simulink model "QuadDynamics"  (R2017b)
settings: Solver=FixedStepAuto  StartTime=0.0  StopTime=10  FixedStep=0.01  RelTol=1e-3
InitFcn:
  | glob
values from neighbouring files (symbols this model uses):
  Earth_g = 9.8    [constant.m]
  UAV_aaa = inv([UAV_kf UAV_kf UAV_kf UAV_kf ... (first row only)    [constant.m]
  UAV_Ixx = 19.688e-3    (= 0.019688)    [constant.m]
  UAV_Iyy = 19.688e-3    (= 0.019688)    [constant.m]
  UAV_Izz = 3.938e-2    (= 0.03938)    [constant.m]
  UAV_kdphi = 0    [constant.m]
  UAV_kdpsai = 0    [constant.m]
  UAV_kdtheta = UAV_kdphi    (= 0)    [constant.m]
  UAV_kdx = 0    [constant.m]
  UAV_kdy = 0    [constant.m]
  UAV_kdz = 0    [constant.m]
  UAV_kipsai = 0    [constant.m]
  UAV_kix = 0    [constant.m]
  UAV_kiy = 0    [constant.m]
  UAV_kiz = 0    [constant.m]
  UAV_kpphi = 0    [constant.m]
  UAV_kppsai = 0    [constant.m]
  UAV_kptheta = UAV_kpphi    (= 0)    [constant.m]
  UAV_kpx = 0    [constant.m]
  UAV_kpy = 0    [constant.m]
  UAV_kpz = 0    [constant.m]
  UAV_L = 0.25    [constant.m]
  UAV_m = 0.75    [constant.m]
  UAV_xf = 3    [constant.m]
  UAV_yf = 4    [constant.m]
  UAV_zf = 5    [constant.m]
settings Model: Creator=root  LastModifiedBy=KingBoy
settings CodeAppCC: StateflowObjectComments=on

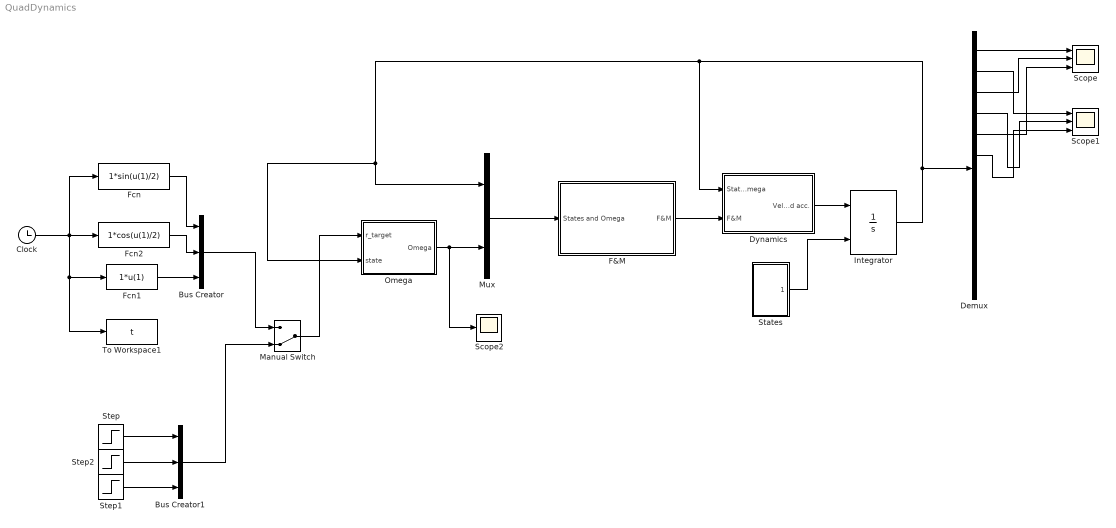
== system QuadDynamics ==
  Bus Creator : BusCreator  Inputs=3
  Bus Creator1 : BusCreator  Inputs=3
  Clock : Clock
  Demux : Demux  Outputs=12
  Dynamics : Subsystem
  F&M : Subsystem
  Fcn : Fcn  Expr=1*sin(u(1)/2)
  Fcn1 : Fcn  Expr=1*u(1)
  Fcn2 : Fcn  Expr=1*cos(u(1)/2)
  Integrator : Integrator  InitialConditionSource=external
  Manual Switch : ManualSwitch  CurrentSetting=0
  Mux : Mux  Inputs=2
  Omega : Subsystem
  Scope : Scope  NumInputPorts=3
  Scope1 : Scope  NumInputPorts=3
  Scope2 : Scope
  States : Subsystem
  Step : Step  Time=0  After=UAV_xf  SampleTime=0
  Step1 : Step  Time=0  After=UAV_zf  SampleTime=0
  Step2 : Step  Time=0  After=UAV_yf  SampleTime=0
  To Workspace1 : ToWorkspace  VariableName=t  SampleTime=-1
      settings: Save2DSignal=2-D array (concatenate along first dimension)
  wires:
  F&M/1(F&M) -> Dynamics/2(F&M)
  Integrator/1 -> Demux/1, Omega/2(state), Mux/1, Dynamics/1(States and Omega)
  Demux/5 -> Scope/3
  States/1("States ") -> Integrator/2
  Omega/1("Omega ") -> Scope2/1, Mux/2
  Mux/1 -> F&M/1(States and Omega)
  Dynamics/1("Velocity and acc. ") -> Integrator/1
  Demux/1 -> Scope/1
  Demux/3 -> Scope/2
  Demux/4 -> Scope1/2
  Demux/6 -> Scope1/3
  Fcn1/1 -> Bus Creator/3
  Clock/1 -> To Workspace1/1, Fcn1/1, Fcn/1, Fcn2/1
  Fcn/1 -> Bus Creator/1
  Fcn2/1 -> Bus Creator/2
  Bus Creator/1 -> Manual Switch/1
  Step2/1 -> Bus Creator1/2
  Step/1 -> Bus Creator1/1
  Bus Creator1/1 -> Manual Switch/2
  Step1/1 -> Bus Creator1/3
  Manual Switch/1 -> Omega/1(r_target)
  Demux/2 -> Scope1/1

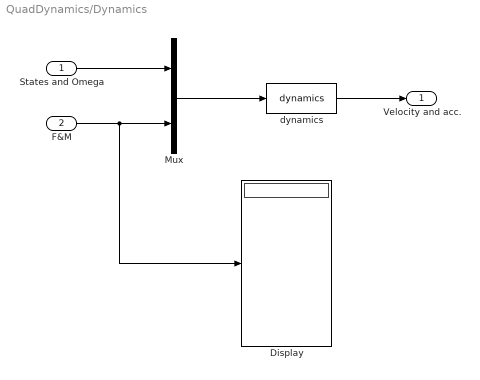
== system QuadDynamics/Dynamics ==
  States and Omega : Inport
  F&M : Inport  Port=2
  Display : Display
  Mux : Mux  Inputs=2
  dynamics : MATLABFcn  MATLABFcn=dynamics  OutputDimensions=12
  "Velocity and acc. " : Outport
  wires:
  Mux/1 -> dynamics/1
  F&M/1 -> Display/1, Mux/2
  States and Omega/1 -> Mux/1
  dynamics/1 -> "Velocity and acc. "/1

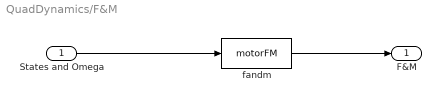
== system QuadDynamics/F&M ==
  States and Omega : Inport
  fandm : MATLABFcn  MATLABFcn=motorFM  OutputDimensions=8
  F&M : Outport
  wires:
  fandm/1 -> F&M/1
  States and Omega/1 -> fandm/1

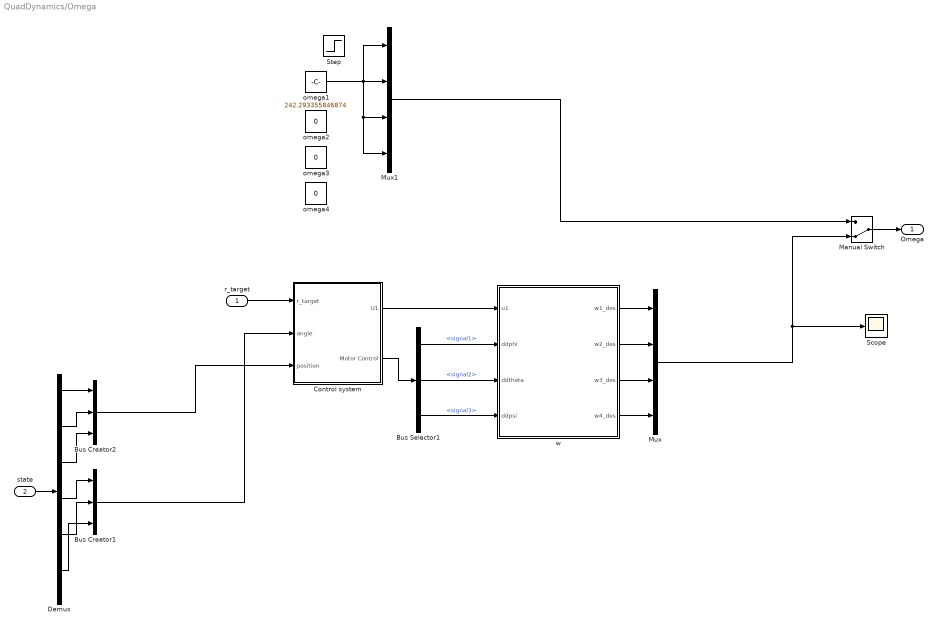
== system QuadDynamics/Omega ==
  r_target : Inport
  state : Inport  Port=2
  Bus Creator1 : BusCreator  Inputs=3
  Bus Creator2 : BusCreator  Inputs=3
  Bus Selector1 : BusSelector  OutputSignals=signal1,signal2,signal3
  Control system : Subsystem
  Demux : Demux  Outputs=12
  Manual Switch : ManualSwitch  CurrentSetting=0
  Mux : Mux
  Mux1 : Mux
  Scope : Scope
  Step : Step  Time=0  After=3  SampleTime=0
  omega1 : Constant  Value=242.293355846874
  omega2 : Constant  Value=0
  omega3 : Constant  Value=0
  omega4 : Constant  Value=0
  w : Subsystem
  "Omega " : Outport
  wires:
  Bus Selector1/3 -> w/4(ddpsi)  "<signal3>"
  Bus Selector1/2 -> w/3(ddtheta)  "<signal2>"
  Bus Selector1/1 -> w/2(ddphi)  "<signal1>"
  Control system/1(U1) -> w/1(u1)
  Control system/2(Motor Control) -> Bus Selector1/1
  w/1(w1_des) -> Mux/1
  w/2(w2_des) -> Mux/2
  w/3(w3_des) -> Mux/3
  w/4(w4_des) -> Mux/4
  r_target/1 -> Control system/1(r_target)
  state/1 -> Demux/1
  Demux/1 -> Bus Creator2/1
  Demux/3 -> Bus Creator2/2
  Demux/5 -> Bus Creator2/3
  Bus Creator2/1 -> Control system/3(position)
  Bus Creator1/1 -> Control system/2(angle)
  Manual Switch/1 -> "Omega "/1
  Mux1/1 -> Manual Switch/1
  Demux/7 -> Bus Creator1/1
  Demux/9 -> Bus Creator1/2
  Demux/11 -> Bus Creator1/3
  Mux/1 -> Scope/1, Manual Switch/2
  omega1/1 -> Mux1/3, Mux1/4, Mux1/2, Mux1/1

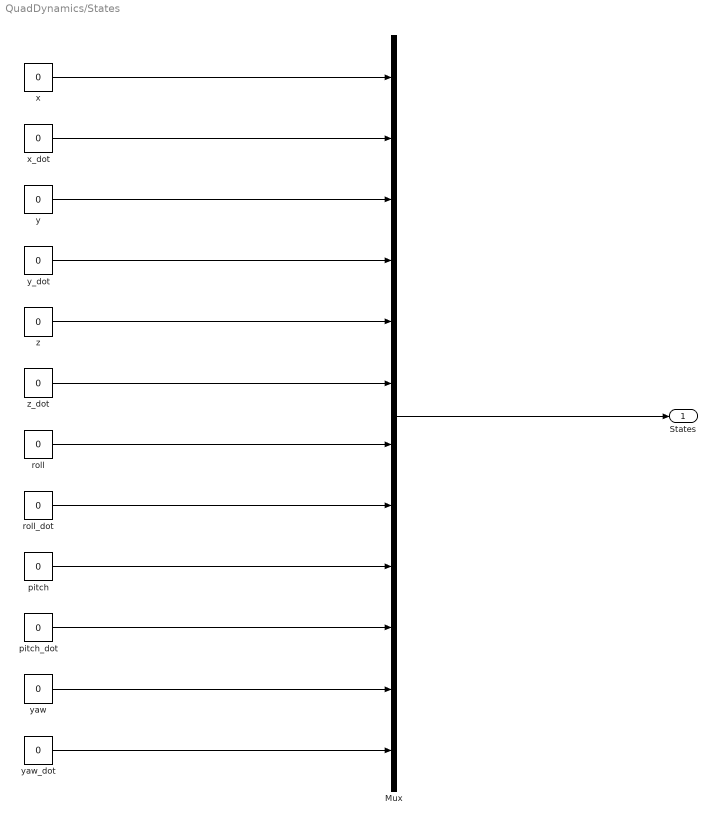
== system QuadDynamics/States ==
  Mux : Mux  Inputs=12
  pitch : Constant  Value=0
  pitch_dot : Constant  Value=0
  roll : Constant  Value=0
  roll_dot : Constant  Value=0
  x : Constant  Value=0
  x_dot : Constant  Value=0
  y : Constant  Value=0
  y_dot : Constant  Value=0
  yaw : Constant  Value=0
  yaw_dot : Constant  Value=0
  z : Constant  Value=0
  z_dot : Constant  Value=0
  "States " : Outport
  wires:
  y/1 -> Mux/3
  z/1 -> Mux/5
  z_dot/1 -> Mux/6
  x/1 -> Mux/1
  pitch_dot/1 -> Mux/10
  x_dot/1 -> Mux/2
  roll/1 -> Mux/7
  yaw/1 -> Mux/11
  y_dot/1 -> Mux/4
  pitch/1 -> Mux/9
  roll_dot/1 -> Mux/8
  yaw_dot/1 -> Mux/12
  Mux/1 -> "States "/1

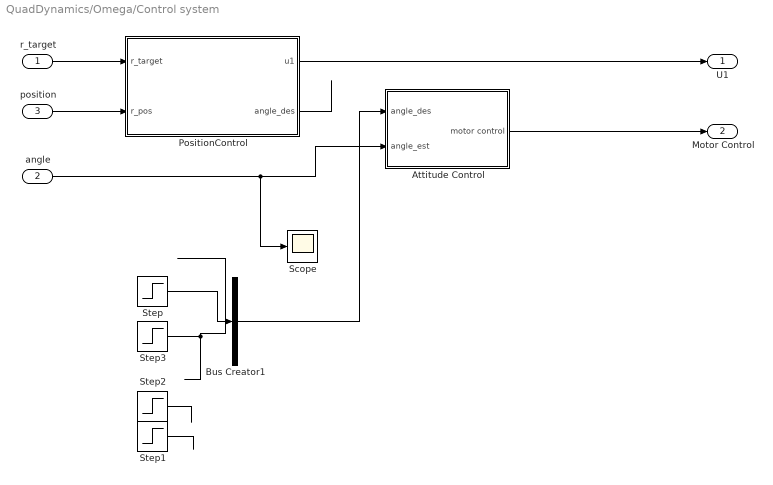
== system QuadDynamics/Omega/Control system ==
  r_target : Inport
  angle : Inport  Port=2
  position : Inport  Port=3
  Attitude Control : Subsystem
  Bus Creator1 : BusCreator  Inputs=3
  PositionControl : Subsystem
  Scope : Scope
  Step : Step  Time=0  After=pi/6  SampleTime=0
  Step1 : Step  Time=0  After=UAV_zf  SampleTime=0
  Step2 : Step  Time=0  After=UAV_yf  SampleTime=0
  Step3 : Step  Time=0  After=0  SampleTime=0
  U1 : Outport
  Motor Control : Outport  Port=2
  wires:
  PositionControl/2(angle_des) -> ?
  angle/1 -> Scope/1, Attitude Control/2(angle_est)
  PositionControl/1(u1) -> U1/1
  Attitude Control/1(motor control) -> Motor Control/1
  position/1 -> PositionControl/2(r_pos)
  r_target/1 -> PositionControl/1(r_target)
  Bus Creator1/1 -> Attitude Control/1(angle_des)
  Step1/1 -> ?
  Step/1 -> Bus Creator1/2
  Step2/1 -> ?
  Step3/1 -> ?

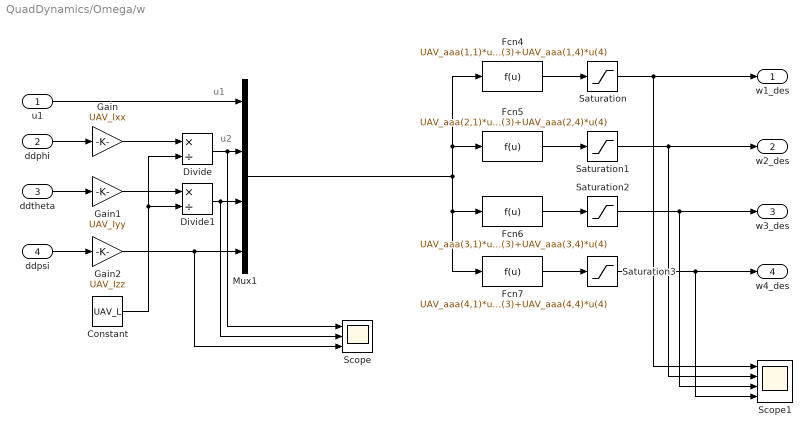
== system QuadDynamics/Omega/w ==
  note: u2
  note: u1
  u1 : Inport
  ddphi : Inport  Port=2
  ddtheta : Inport  Port=3
  ddpsi : Inport  Port=4
  Constant : Constant  Value=UAV_L
  Divide : Product  Inputs=*/
  Divide1 : Product  Inputs=*/
  Fcn4 : Fcn  Expr=UAV_aaa(1,1)*u(1)+UAV_aaa(1,2)*u(2)+UAV_aaa(1,3)*u(3)+UAV_aaa(1,4)*u(4)
  Fcn5 : Fcn  Expr=UAV_aaa(2,1)*u(1)+UAV_aaa(2,2)*u(2)+UAV_aaa(2,3)*u(3)+UAV_aaa(2,4)*u(4)
  Fcn6 : Fcn  Expr=UAV_aaa(3,1)*u(1)+UAV_aaa(3,2)*u(2)+UAV_aaa(3,3)*u(3)+UAV_aaa(3,4)*u(4)
  Fcn7 : Fcn  Expr=UAV_aaa(4,1)*u(1)+UAV_aaa(4,2)*u(2)+UAV_aaa(4,3)*u(3)+UAV_aaa(4,4)*u(4)
  Gain : Gain  Gain=UAV_Ixx
  Gain1 : Gain  Gain=UAV_Iyy
  Gain2 : Gain  Gain=UAV_Izz
  Mux1 : Mux
  Saturation{,1..3} (4 alike) : Saturate  UpperLimit=(9000*2*pi/60)^2  LowerLimit=0
  Scope : Scope  NumInputPorts=3
  Scope1 : Scope  NumInputPorts=4
  w1_des : Outport
  w2_des : Outport  Port=2
  w3_des : Outport  Port=3
  w4_des : Outport  Port=4
  wires:
  u1/1 -> Mux1/1
  ddphi/1 -> Gain/1
  ddpsi/1 -> Gain2/1
  ddtheta/1 -> Gain1/1
  Fcn4/1 -> Saturation/1
  Fcn6/1 -> Saturation2/1
  Fcn7/1 -> Saturation3/1
  Saturation/1 -> Scope1/1, w1_des/1
  Saturation1/1 -> Scope1/2, w2_des/1
  Saturation2/1 -> Scope1/3, w3_des/1
  Saturation3/1 -> Scope1/4, w4_des/1
  Divide/1 -> Scope/1, Mux1/2
  Gain/1 -> Divide/1
  Constant/1 -> Divide1/2, Divide/2
  Divide1/1 -> Scope/2, Mux1/3
  Gain2/1 -> Scope/3, Mux1/4
  Gain1/1 -> Divide1/1
  Fcn5/1 -> Saturation1/1
  Mux1/1 -> Fcn7/1, Fcn6/1, Fcn5/1, Fcn4/1

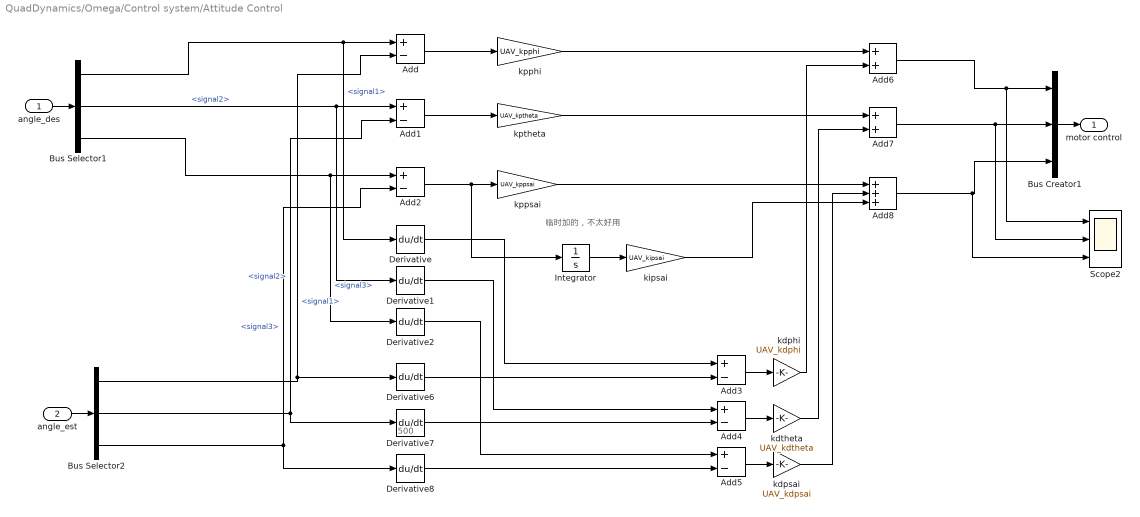
== system QuadDynamics/Omega/Control system/Attitude Control ==
  note: 临时加的，不太好用
  note: 500
  angle_des : Inport
  angle_est : Inport  Port=2
  Add{,1..5} (6 alike) : Sum  Inputs=+-
  Add6 : Sum
  Add7 : Sum
  Add8 : Sum  Inputs=+++
  Bus Creator1 : BusCreator  Inputs=3
  Bus Selector1 : BusSelector  OutputSignals=signal1,signal2,signal3
  Bus Selector2 : BusSelector  OutputSignals=signal1,signal2,signal3
  Derivative{,1..2,6..8} (6 alike) : Derivative  CoefficientInTFapproximation=500
  Integrator : Integrator
  Scope2 : Scope  NumInputPorts=3
  kdphi : Gain  Gain=UAV_kdphi
  kdpsai : Gain  Gain=UAV_kdpsai
  kdtheta : Gain  Gain=UAV_kdtheta
  kipsai : Gain  Gain=UAV_kipsai
  kpphi : Gain  Gain=UAV_kpphi
  kppsai : Gain  Gain=UAV_kppsai
  kptheta : Gain  Gain=UAV_kptheta
  motor control : Outport
  wires:
  Bus Selector1/1 -> Add/1, Derivative/1  "<signal1>"
  Bus Selector2/1 -> Add/2, Derivative6/1  "<signal1>"
  Add/1 -> kpphi/1
  Bus Selector1/2 -> Derivative1/1, Add1/1  "<signal2>"
  Bus Selector2/2 -> Add1/2, Derivative7/1  "<signal2>"
  Add1/1 -> kptheta/1
  Add2/1 -> Integrator/1, kppsai/1
  Bus Selector1/3 -> Derivative2/1, Add2/1  "<signal3>"
  Bus Selector2/3 -> Add2/2, Derivative8/1  "<signal3>"
  Add3/1 -> kdphi/1
  Add4/1 -> kdtheta/1
  Add5/1 -> kdpsai/1
  kpphi/1 -> Add6/1
  kdphi/1 -> Add6/2
  kptheta/1 -> Add7/1
  kdtheta/1 -> Add7/2
  kppsai/1 -> Add8/1
  kdpsai/1 -> Add8/2
  Derivative/1 -> Add3/1
  Derivative1/1 -> Add4/1
  Derivative2/1 -> Add5/1
  Derivative6/1 -> Add3/2
  Derivative7/1 -> Add4/2
  Derivative8/1 -> Add5/2
  angle_est/1 -> Bus Selector2/1
  angle_des/1 -> Bus Selector1/1
  Bus Creator1/1 -> motor control/1
  Add6/1 -> Scope2/1, Bus Creator1/1
  Add7/1 -> Scope2/2, Bus Creator1/2
  Add8/1 -> Scope2/3, Bus Creator1/3
  Integrator/1 -> kipsai/1
  kipsai/1 -> Add8/3

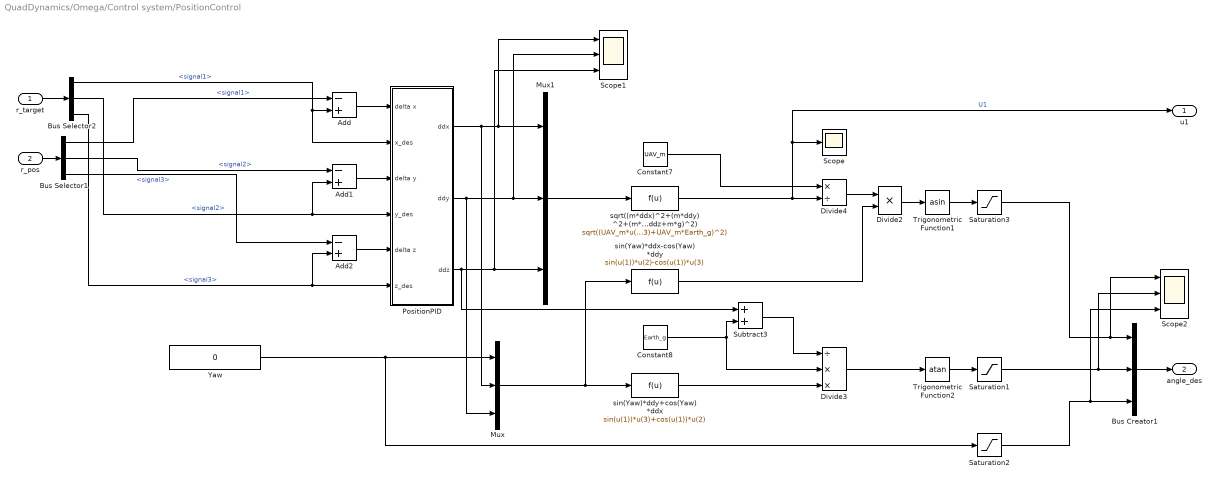
== system QuadDynamics/Omega/Control system/PositionControl ==
  r_target : Inport
  r_pos : Inport  Port=2
  Add : Sum  Inputs=-+
  Add1 : Sum  Inputs=-+
  Add2 : Sum  Inputs=-+
  Bus Creator1 : BusCreator  Inputs=3
  Bus Selector1 : BusSelector  OutputSignals=signal1,signal2,signal3
  Bus Selector2 : BusSelector  OutputSignals=signal1,signal2,signal3
  Constant7 : Constant  Value=UAV_m
  Constant8 : Constant  Value=Earth_g
  Divide2 : Product  Inputs=**
  Divide3 : Product  Inputs=/**
  Divide4 : Product  Inputs=*/
  Mux : Mux  Inputs=3
  Mux1 : Mux  Inputs=3
  PositionPID : Subsystem
  Saturation1 : Saturate  UpperLimit=90/57.3  LowerLimit=-90/57.3
  Saturation2 : Saturate  UpperLimit=90/57.3  LowerLimit=-90/57.3
  Saturation3 : Saturate  UpperLimit=90/57.3  LowerLimit=-90/57.3
  Scope : Scope
  Scope1 : Scope  NumInputPorts=3
  Scope2 : Scope  NumInputPorts=3
  Subtract3 : Sum
  Trigonometric Function1 : Trigonometry  Operator=asin
  Trigonometric Function2 : Trigonometry  Operator=atan
  Yaw : Constant  Value=0
  sin(Yaw)*ddx-cos(Yaw)*ddy : Fcn  Expr=sin(u(1))*u(2)-cos(u(1))*u(3)
  sin(Yaw)*ddy+cos(Yaw)*ddx : Fcn  Expr=sin(u(1))*u(3)+cos(u(1))*u(2)
  sqrt((m*ddx)^2+(m*ddy)^2+(m*ddz+m*g)^2) : Fcn  Expr=sqrt((UAV_m*u(1))^2+(UAV_m*u(2))^2+(UAV_m*u(3)+UAV_m*Earth_g)^2)
  u1 : Outport
  angle_des : Outport  Port=2
  wires:
  Bus Selector1/1 -> Add/1  "<signal1>"
  Add/1 -> PositionPID/1(delta x)
  Bus Selector1/2 -> Add1/1  "<signal2>"
  Bus Selector2/2 -> Add1/2, PositionPID/4(y_des)  "<signal2>"
  Add1/1 -> PositionPID/3(delta y)
  Bus Selector1/3 -> Add2/1  "<signal3>"
  Bus Selector2/3 -> Add2/2, PositionPID/6(z_des)  "<signal3>"
  Add2/1 -> PositionPID/5(delta z)
  PositionPID/2(ddy) -> Mux/3, Scope1/2, Mux1/2
  sqrt((m*ddx)^2+(m*ddy)^2+(m*ddz+m*g)^2)/1 -> u1/1, Scope/1, Divide4/2  "U1"
  PositionPID/3(ddz) -> Subtract3/1, Scope1/3, Mux1/3
  sin(Yaw)*ddx-cos(Yaw)*ddy/1 -> Divide2/2
  Divide3/1 -> Trigonometric Function2/1
  Constant7/1 -> Divide4/1
  Divide4/1 -> Divide2/1
  Constant8/1 -> Divide3/2, Subtract3/2
  Trigonometric Function2/1 -> Saturation1/1
  Trigonometric Function1/1 -> Saturation3/1
  Divide2/1 -> Trigonometric Function1/1
  PositionPID/1(ddx) -> Scope1/1, Mux1/1, Mux/2
  Yaw/1 -> Mux/1, Saturation2/1
  Subtract3/1 -> Divide3/1
  Saturation3/1 -> Scope2/1, Bus Creator1/1
  Saturation1/1 -> Scope2/2, Bus Creator1/2
  Saturation2/1 -> Scope2/3, Bus Creator1/3
  Mux/1 -> sin(Yaw)*ddx-cos(Yaw)*ddy/1, sin(Yaw)*ddy+cos(Yaw)*ddx/1
  Mux1/1 -> sqrt((m*ddx)^2+(m*ddy)^2+(m*ddz+m*g)^2)/1
  sin(Yaw)*ddy+cos(Yaw)*ddx/1 -> Divide3/3
  r_pos/1 -> Bus Selector1/1
  r_target/1 -> Bus Selector2/1
  Bus Selector2/1 -> PositionPID/2(x_des), Add/2  "<signal1>"
  Bus Creator1/1 -> angle_des/1

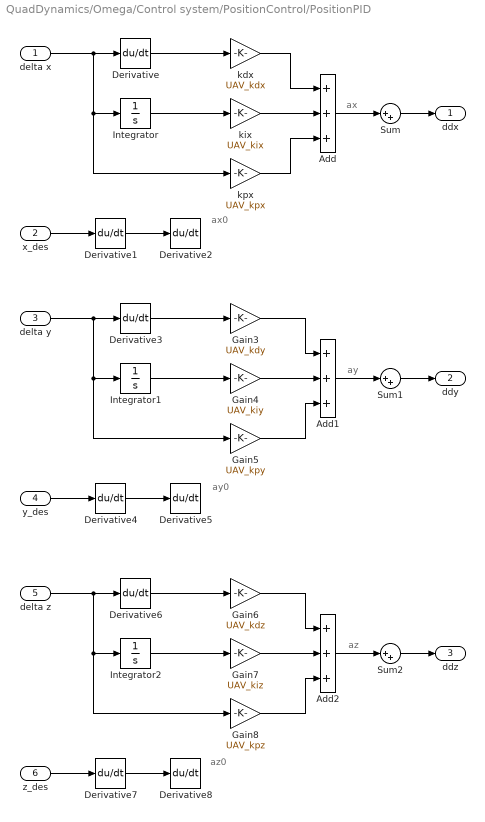
== system QuadDynamics/Omega/Control system/PositionControl/PositionPID ==
  note: az
  note: ay
  note: ax
  note: az0
  note: ay0
  note: ax0
  delta x : Inport
  x_des : Inport  Port=2
  delta y : Inport  Port=3
  y_des : Inport  Port=4
  delta z : Inport  Port=5
  z_des : Inport  Port=6
  Add : Sum  Inputs=+++
  Add1 : Sum  Inputs=+++
  Add2 : Sum  Inputs=+++
  Derivative{,1..5,7..8} (8 alike) : Derivative  CoefficientInTFapproximation=500
  Derivative6 : Derivative
  Gain3 : Gain  Gain=UAV_kdy
  Gain4 : Gain  Gain=UAV_kiy
  Gain5 : Gain  Gain=UAV_kpy
  Gain6 : Gain  Gain=UAV_kdz
  Gain7 : Gain  Gain=UAV_kiz
  Gain8 : Gain  Gain=UAV_kpz
  Integrator : Integrator
  Integrator1 : Integrator
  Integrator2 : Integrator
  Sum : Sum  Inputs=|++
  Sum1 : Sum  Inputs=|++
  Sum2 : Sum  Inputs=|++
  kdx : Gain  Gain=UAV_kdx
  kix : Gain  Gain=UAV_kix
  kpx : Gain  Gain=UAV_kpx
  ddx : Outport
  ddy : Outport  Port=2
  ddz : Outport  Port=3
  wires:
  delta x/1 -> kpx/1, Integrator/1, Derivative/1
  Derivative/1 -> kdx/1
  kdx/1 -> Add/1
  Integrator/1 -> kix/1
  kix/1 -> Add/2
  kpx/1 -> Add/3
  Add/1 -> Sum/1
  Derivative1/1 -> Derivative2/1
  x_des/1 -> Derivative1/1
  Sum/1 -> ddx/1
  delta y/1 -> Gain5/1, Integrator1/1, Derivative3/1
  Derivative3/1 -> Gain3/1
  Gain3/1 -> Add1/1
  Integrator1/1 -> Gain4/1
  Gain4/1 -> Add1/2
  Gain5/1 -> Add1/3
  Add1/1 -> Sum1/1
  Derivative4/1 -> Derivative5/1
  y_des/1 -> Derivative4/1
  Sum1/1 -> ddy/1
  delta z/1 -> Gain8/1, Integrator2/1, Derivative6/1
  Derivative6/1 -> Gain6/1
  Gain6/1 -> Add2/1
  Integrator2/1 -> Gain7/1
  Gain7/1 -> Add2/2
  Gain8/1 -> Add2/3
  Add2/1 -> Sum2/1
  Derivative7/1 -> Derivative8/1
  z_des/1 -> Derivative7/1
  Sum2/1 -> ddz/1
